simulink model "DIT8FFT"  (Simulink 6.3)
settings: Solver=FixedStepDiscrete  StartTime=0.0  StopTime=5  FixedStep=1  RelTol=1e-3
InitFcn:
  | %% DSPBuilder Start
  | alt_dspbuilder_update_model(bdroot)
  | %% DSPBuilder End
libraries: allblocks_alteradspbuilder2 x56
settings Model: LastModifiedBy=LKONG  StrictBusMsg=None
settings DataIOCC: SignalLoggingName=sigsOut
settings OptimizationCC: BooleanDataType=off  InlineInvariantSignals=on
settings DebuggingCC: SolverPrmCheckMsg=none
settings HardwareCC: TargetUnknown=on

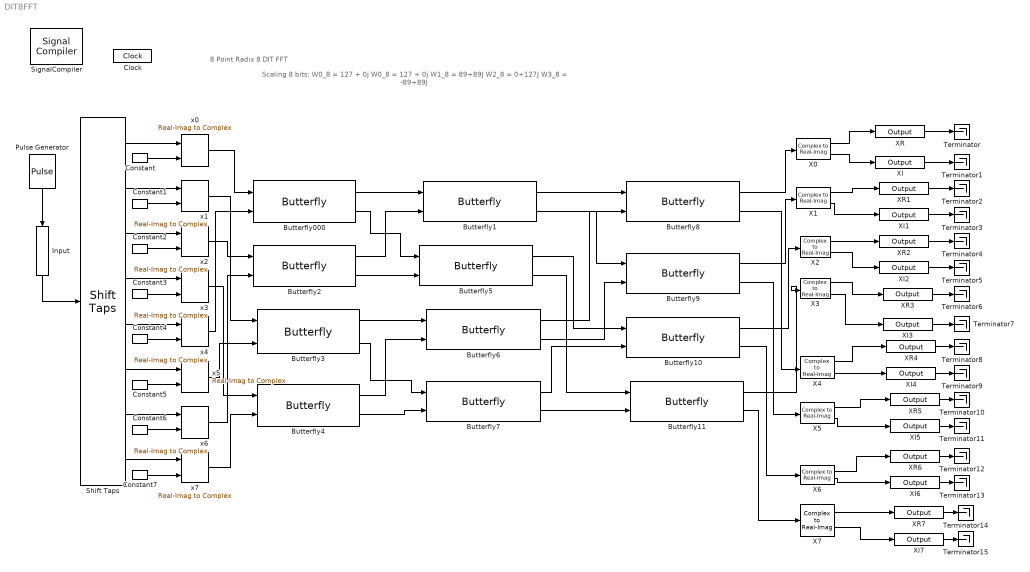
== system DIT8FFT ==
  note: 8 Point Radix 8 DIT FFT
  note: Scaling 8 bits:
      | W0_8 = 127 + 0j
      | W0_8 = 127 + 0j
      | W1_8 = 89+89J
      | W2_8 = 0+127J
      | W3_8 = -89+89J
  Butterfly000 : allblocks_alteradspbuilder2/Butterfly  BusType=Signed Integer  ibwl=8  ibwr=0  pipeline=5  full_resolution=off  obwl=9  obwr=0  olsb=8  constant_W=on  W_real=127  W_imag=0  dedicated_circuitry=Auto  use_ena=off  use_aclr=off
  Butterfly1 : allblocks_alteradspbuilder2/Butterfly  BusType=Signed Integer  ibwl=9  ibwr=0  pipeline=5  full_resolution=off  obwl=10  obwr=0  olsb=8  constant_W=on  W_real=127  W_imag=0  dedicated_circuitry=Auto  use_ena=off  use_aclr=off
  Butterfly10 : allblocks_alteradspbuilder2/Butterfly  BusType=Signed Integer  ibwl=10  ibwr=0  pipeline=5  full_resolution=off  obwl=11  obwr=0  olsb=10  constant_W=on  W_real=0  W_imag=127  dedicated_circuitry=Auto  use_ena=off  use_aclr=off
  Butterfly11 : allblocks_alteradspbuilder2/Butterfly  BusType=Signed Integer  ibwl=10  ibwr=0  pipeline=5  full_resolution=off  obwl=11  obwr=0  olsb=10  constant_W=on  W_real=-89  W_imag=89  dedicated_circuitry=Auto  use_ena=off  use_aclr=off
  Butterfly2 : allblocks_alteradspbuilder2/Butterfly  BusType=Signed Integer  ibwl=8  ibwr=0  pipeline=5  full_resolution=off  obwl=9  obwr=0  olsb=8  constant_W=on  W_real=127  W_imag=0  dedicated_circuitry=Auto  use_ena=off  use_aclr=off
  Butterfly3 : allblocks_alteradspbuilder2/Butterfly  BusType=Signed Integer  ibwl=8  ibwr=0  pipeline=5  full_resolution=off  obwl=9  obwr=0  olsb=8  constant_W=on  W_real=127  W_imag=0  dedicated_circuitry=Auto  use_ena=off  use_aclr=off
  Butterfly4 : allblocks_alteradspbuilder2/Butterfly  BusType=Signed Integer  ibwl=8  ibwr=0  pipeline=5  full_resolution=off  obwl=9  obwr=0  olsb=8  constant_W=on  W_real=127  W_imag=0  dedicated_circuitry=Auto  use_ena=off  use_aclr=off
  Butterfly5 : allblocks_alteradspbuilder2/Butterfly  BusType=Signed Integer  ibwl=9  ibwr=0  pipeline=5  full_resolution=off  obwl=10  obwr=0  olsb=8  constant_W=on  W_real=127  W_imag=0  dedicated_circuitry=Auto  use_ena=off  use_aclr=off
  Butterfly6 : allblocks_alteradspbuilder2/Butterfly  BusType=Signed Integer  ibwl=9  ibwr=0  pipeline=5  full_resolution=off  obwl=10  obwr=0  olsb=8  constant_W=on  W_real=0  W_imag=127  dedicated_circuitry=Auto  use_ena=off  use_aclr=off
  Butterfly7 : allblocks_alteradspbuilder2/Butterfly  BusType=Signed Integer  ibwl=9  ibwr=0  pipeline=5  full_resolution=off  obwl=10  obwr=0  olsb=8  constant_W=on  W_real=0  W_imag=127  dedicated_circuitry=Auto  use_ena=off  use_aclr=off
  Butterfly8 : allblocks_alteradspbuilder2/Butterfly  BusType=Signed Integer  ibwl=10  ibwr=0  pipeline=5  full_resolution=off  obwl=11  obwr=0  olsb=10  constant_W=on  W_real=127  W_imag=0  dedicated_circuitry=Auto  use_ena=off  use_aclr=off
  Butterfly9 : allblocks_alteradspbuilder2/Butterfly  BusType=Signed Integer  ibwl=10  ibwr=0  pipeline=5  full_resolution=off  obwl=11  obwr=0  olsb=10  constant_W=on  W_real=89  W_imag=89  dedicated_circuitry=Auto  use_ena=off  use_aclr=off
  Clock : allblocks_alteradspbuilder2/Clock  ClockPeriod=100  ClockPeriodUnit=ns  SampleTime=1  SimulationStartCycle=5  PhaseOffset=0  Reset=aclr  Export=off
  Constant{,1..7} (8 alike) : allblocks_alteradspbuilder2/Constant  mask_cst=0  BusType=Signed Integer  bwl=8  bwr=0  SpecifyClock=off
  Input : allblocks_alteradspbuilder2/Input  Orientation=down  iofile=D:\dspbuilder\dspb_71\DesignExamples\demos\Transforms\8PointFFT\tb_DIT8FFT\DIT8FFT_Input.salt  BusType=Signed Integer  bwl=8  bwr=0  SpecifyClock=off  PORTTYPE=Input
  Pulse Generator : DiscretePulseGenerator  Orientation=down  PulseType=Time based  PulseWidth=50
  Shift Taps : allblocks_alteradspbuilder2/Shift Taps  number_of_taps=8  tap_distance=1  use_shiftout=off  use_ena=off  use_sclr=off  use_dedicated_circuitry=on  ram_type=AUTO
  SignalCompiler : allblocks_alteradspbuilder2/Signal Compiler  DeviceFamily=Stratix IV  DeviceName=AUTO  EnableSignalTap=off  SignalTapDepth=128  UseBoardBlock=off  StpUseDefaultClock=on  StpClock=Clock
  Terminator{,1..15} (16 alike) : Terminator
  X{0..7} (8 alike) : allblocks_alteradspbuilder2/Complex to Real-Imag  BusType=Signed Integer  bwl=11  bwr=0
  XI : allblocks_alteradspbuilder2/Output  iofile=D:\dspbuilder\dspb_71\DesignExamples\demos\Transforms\8PointFFT\tb_DIT8FFT\DIT8FFT_XI.capture  BusType=Signed Integer  bwl=16  bwr=0  PORTTYPE=Output
  XI1 : allblocks_alteradspbuilder2/Output  iofile=D:\dspbuilder\dspb_71\DesignExamples\demos\Transforms\8PointFFT\tb_DIT8FFT\DIT8FFT_XI1.capture  BusType=Signed Integer  bwl=16  bwr=0  PORTTYPE=Output
  XI2 : allblocks_alteradspbuilder2/Output  iofile=D:\dspbuilder\dspb_71\DesignExamples\demos\Transforms\8PointFFT\tb_DIT8FFT\DIT8FFT_XI2.capture  BusType=Signed Integer  bwl=16  bwr=0  PORTTYPE=Output
  XI3 : allblocks_alteradspbuilder2/Output  iofile=D:\dspbuilder\dspb_71\DesignExamples\demos\Transforms\8PointFFT\tb_DIT8FFT\DIT8FFT_XI3.capture  BusType=Signed Integer  bwl=16  bwr=0  PORTTYPE=Output
  XI4 : allblocks_alteradspbuilder2/Output  iofile=D:\dspbuilder\dspb_71\DesignExamples\demos\Transforms\8PointFFT\tb_DIT8FFT\DIT8FFT_XI4.capture  BusType=Signed Integer  bwl=16  bwr=0  PORTTYPE=Output
  XI5 : allblocks_alteradspbuilder2/Output  iofile=D:\dspbuilder\dspb_71\DesignExamples\demos\Transforms\8PointFFT\tb_DIT8FFT\DIT8FFT_XI5.capture  BusType=Signed Integer  bwl=16  bwr=0  PORTTYPE=Output
  XI6 : allblocks_alteradspbuilder2/Output  iofile=D:\dspbuilder\dspb_71\DesignExamples\demos\Transforms\8PointFFT\tb_DIT8FFT\DIT8FFT_XI6.capture  BusType=Signed Integer  bwl=16  bwr=0  PORTTYPE=Output
  XI7 : allblocks_alteradspbuilder2/Output  iofile=D:\dspbuilder\dspb_71\DesignExamples\demos\Transforms\8PointFFT\tb_DIT8FFT\DIT8FFT_XI7.capture  BusType=Signed Integer  bwl=16  bwr=0  PORTTYPE=Output
  XR : allblocks_alteradspbuilder2/Output  iofile=D:\dspbuilder\dspb_71\DesignExamples\demos\Transforms\8PointFFT\tb_DIT8FFT\DIT8FFT_XR.capture  BusType=Signed Integer  bwl=16  bwr=0  PORTTYPE=Output
  XR1 : allblocks_alteradspbuilder2/Output  iofile=D:\dspbuilder\dspb_71\DesignExamples\demos\Transforms\8PointFFT\tb_DIT8FFT\DIT8FFT_XR1.capture  BusType=Signed Integer  bwl=16  bwr=0  PORTTYPE=Output
  XR2 : allblocks_alteradspbuilder2/Output  iofile=D:\dspbuilder\dspb_71\DesignExamples\demos\Transforms\8PointFFT\tb_DIT8FFT\DIT8FFT_XR2.capture  BusType=Signed Integer  bwl=16  bwr=0  PORTTYPE=Output
  XR3 : allblocks_alteradspbuilder2/Output  iofile=D:\dspbuilder\dspb_71\DesignExamples\demos\Transforms\8PointFFT\tb_DIT8FFT\DIT8FFT_XR3.capture  BusType=Signed Integer  bwl=16  bwr=0  PORTTYPE=Output
  XR4 : allblocks_alteradspbuilder2/Output  iofile=D:\dspbuilder\dspb_71\DesignExamples\demos\Transforms\8PointFFT\tb_DIT8FFT\DIT8FFT_XR4.capture  BusType=Signed Integer  bwl=16  bwr=0  PORTTYPE=Output
  XR5 : allblocks_alteradspbuilder2/Output  iofile=D:\dspbuilder\dspb_71\DesignExamples\demos\Transforms\8PointFFT\tb_DIT8FFT\DIT8FFT_XR5.capture  BusType=Signed Integer  bwl=16  bwr=0  PORTTYPE=Output
  XR6 : allblocks_alteradspbuilder2/Output  iofile=D:\dspbuilder\dspb_71\DesignExamples\demos\Transforms\8PointFFT\tb_DIT8FFT\DIT8FFT_XR6.capture  BusType=Signed Integer  bwl=16  bwr=0  PORTTYPE=Output
  XR7 : allblocks_alteradspbuilder2/Output  iofile=D:\dspbuilder\dspb_71\DesignExamples\demos\Transforms\8PointFFT\tb_DIT8FFT\DIT8FFT_XR7.capture  BusType=Signed Integer  bwl=16  bwr=0  PORTTYPE=Output
  x{0..7} (8 alike) : allblocks_alteradspbuilder2/Real-Imag to Complex  BusType=Signed Integer  bwl=8  bwr=0
  wires:
  Constant/1 -> x0/2
  Constant1/1 -> x1/2
  Constant2/1 -> x2/2
  Constant3/1 -> x3/2
  Constant4/1 -> x4/2
  Constant5/1 -> x5/2
  Constant6/1 -> x6/2
  Constant7/1 -> x7/2
  Shift Taps/1 -> x0/1
  Shift Taps/2 -> x1/1
  Shift Taps/3 -> x2/1
  Shift Taps/4 -> x3/1
  Shift Taps/5 -> x4/1
  Shift Taps/6 -> x5/1
  Shift Taps/7 -> x6/1
  Shift Taps/8 -> x7/1
  Input/1 -> Shift Taps/1
  x0/1 -> Butterfly000/1
  x3/1 -> Butterfly4/1
  x4/1 -> Butterfly000/2
  x7/1 -> Butterfly4/2
  Butterfly1/1 -> Butterfly8/1
  Butterfly000/1 -> Butterfly1/1
  X0/1 -> XR/1
  X0/2 -> XI/1
  X1/1 -> XR1/1
  X1/2 -> XI1/1
  X2/1 -> XR2/1
  X2/2 -> XI2/1
  X3/1 -> XR3/1
  X3/2 -> XI3/1
  X4/1 -> XR4/1
  X4/2 -> XI4/1
  X5/1 -> XR5/1
  X5/2 -> XI5/1
  X6/1 -> XR6/1
  X6/2 -> XI6/1
  X7/1 -> XR7/1
  X7/2 -> XI7/1
  x2/1 -> Butterfly2/1
  x1/1 -> Butterfly3/1
  x5/1 -> Butterfly3/2
  Butterfly2/1 -> Butterfly1/2
  Butterfly000/2 -> Butterfly5/1
  Butterfly2/2 -> Butterfly5/2
  Butterfly3/1 -> Butterfly6/1
  Butterfly4/1 -> Butterfly6/2
  Butterfly4/2 -> Butterfly7/2
  Butterfly3/2 -> Butterfly7/1
  Butterfly6/1 -> Butterfly8/2
  Butterfly1/2 -> Butterfly9/1
  Butterfly6/2 -> Butterfly9/2
  Butterfly5/1 -> Butterfly10/1
  Butterfly7/1 -> Butterfly10/2
  Butterfly5/2 -> Butterfly11/1
  Butterfly7/2 -> Butterfly11/2
  Butterfly8/1 -> X0/1
  Butterfly9/1 -> X1/1
  Butterfly10/1 -> X2/1
  Butterfly11/1 -> X3/1
  Butterfly8/2 -> X4/1
  Butterfly9/2 -> X5/1
  Butterfly10/2 -> X6/1
  Butterfly11/2 -> X7/1
  x6/1 -> Butterfly2/2
  XR/1 -> Terminator/1
  XI/1 -> Terminator1/1
  XR1/1 -> Terminator2/1
  XI1/1 -> Terminator3/1
  XR2/1 -> Terminator4/1
  XI2/1 -> Terminator5/1
  XR3/1 -> Terminator6/1
  XI3/1 -> Terminator7/1
  XR4/1 -> Terminator8/1
  XI4/1 -> Terminator9/1
  XR5/1 -> Terminator10/1
  XI5/1 -> Terminator11/1
  XR6/1 -> Terminator12/1
  XI6/1 -> Terminator13/1
  XR7/1 -> Terminator14/1
  XI7/1 -> Terminator15/1
  Pulse Generator/1 -> Input/1
